simulink model "W06_P3_boat_speed"  (R2024b)
settings: Solver=ode4  StartTime=0.0  StopTime=60  FixedStep=0.01  RelTol=1e-3
values from neighbouring files (symbols this model uses):
  Kb_u = 2    [W06_pid_setup.m]
  Kd_u = 0    [W06_pid_setup.m]
  Ki_u = 300    [W06_pid_setup.m]    (also in W06_setup.m = 100; W08_setup.m = 100)
  Kp_u = 300    [W06_pid_setup.m]    (also in W06_setup.m; W08_setup.m)
  Nf_u = 20    [W06_pid_setup.m]
  tau_m = 0.30    (= 0.3)    [W06_pid_setup.m]
  X_max = 500    [W06_pid_setup.m]
settings Model: Creator=admin  LastModifiedBy=admin

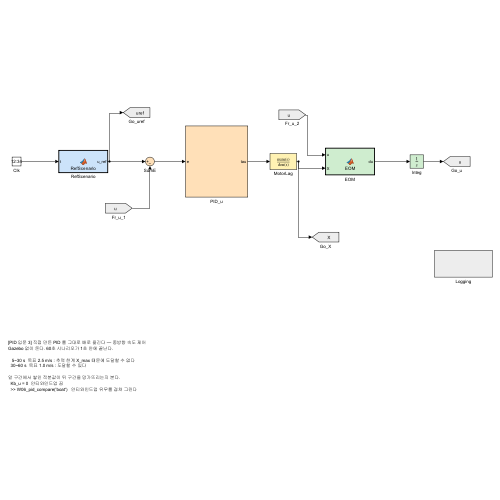
[thumbnail: Simulink's stored preview of the top-level diagram]
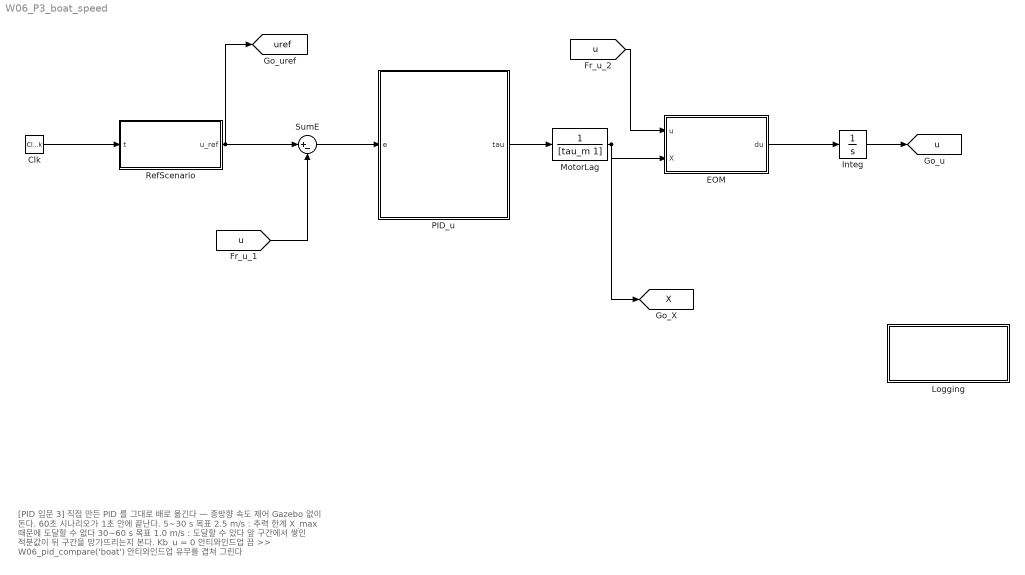
== system W06_P3_boat_speed ==
  note: [PID 입문 3] 직접 만든 PID 를 그대로 배로 옮긴다 — 종방향 속도 제어
      | Gazebo 없이 돈다. 60초 시나리오가 1초 안에 끝난다.
      |
      |    5~30 s  목표 2.5 m/s : 추력 한계 X_max 때문에 도달할 수 없다
      |   30~60 s  목표 1.0 m/s : 도달할 수 있다
      |
      | 앞 구간에서 쌓인 적분값이 뒤 구간을 망가뜨리는지 본다.
      |   Kb_u = 0  안티와인드업 끔
      |   >> W06_pid_compare('boat')   안티와인드업 유무를 겹쳐 그린다
  Clk : DigitalClock  SampleTime=0.01
  EOM : MATLAB Function  TreatAsAtomicUnit=on
  Integ : Integrator
  Logging : Subsystem
  MotorLag : TransferFcn  Numerator=1  Denominator=[tau_m 1]
  PID_u : Subsystem
  RefScenario : MATLAB Function  TreatAsAtomicUnit=on
  SumE : Sum  Inputs=|+-
  tag scope: X=global, u=global, uref=global
  wires:
  Clk/1 -> RefScenario/1(t)
  RefScenario/1(u_ref) -> SumE/1, [uref]
  SumE/1 -> PID_u/1(e)
  PID_u/1(tau) -> MotorLag/1
  EOM/1(du) -> Integ/1
  Integ/1 -> [u]
  MotorLag/1 -> EOM/2(X), [X]
  [u] -> EOM/1(u)
  [u] -> SumE/2

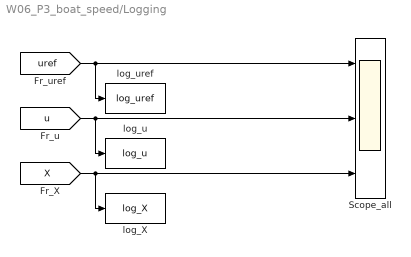
== system W06_P3_boat_speed/Logging ==
  Scope_all : Scope  NumInputPorts=3
  log_X : ToWorkspace  VariableName=log_X  SaveFormat=Timeseries  SampleTime=-1
  log_u : ToWorkspace  VariableName=log_u  SaveFormat=Timeseries  SampleTime=-1
  log_uref : ToWorkspace  VariableName=log_uref  SaveFormat=Timeseries  SampleTime=-1
  wires:
  [uref] -> Scope_all/1, log_uref/1
  [u] -> Scope_all/2, log_u/1
  [X] -> Scope_all/3, log_X/1

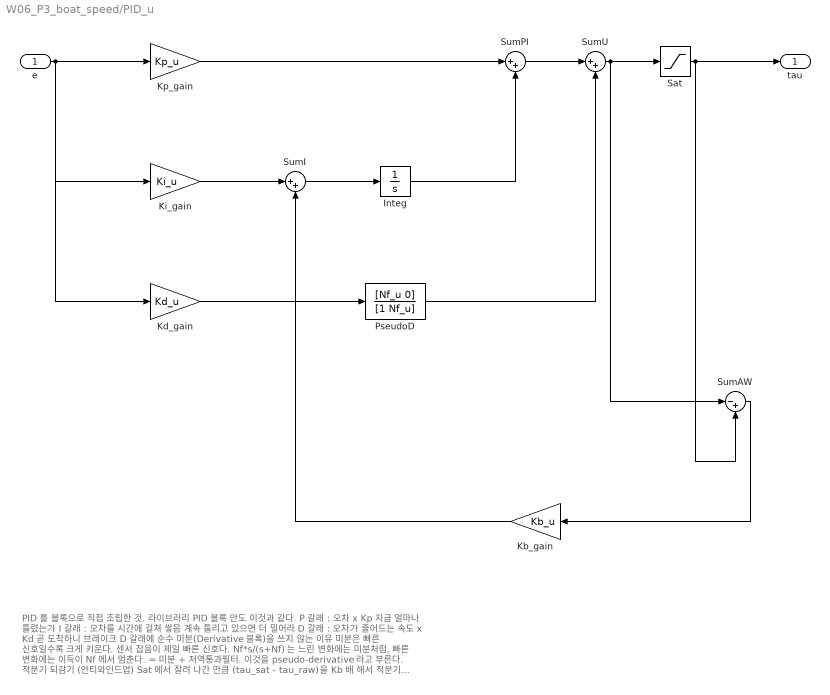
== system W06_P3_boat_speed/PID_u ==
  note: PID 를 블록으로 직접 조립한 것. 라이브러리 PID 블록 안도 이것과 같다.
      |
      |   P 갈래  : 오차 x Kp                        지금 얼마나 틀렸는가
      |   I 갈래  : 오차를 시간에 걸쳐 쌓음            계속 틀리고 있으면 더 밀어라
      |   D 갈래  : 오차가 줄어드는 속도 x Kd          곧 도착하니 브레이크
      |
      | D 갈래에 순수 미분(Derivative 블록)을 쓰지 않는 이유
      |   미분은 빠른 신호일수록 크게 키운다. 센서 잡음이 제일 빠른 신호다.
      |   Nf*s/(s+Nf) 는 느린 변화에는 미분처럼, 빠른 변화에는 이득이 Nf 에서 멈춘다.
      |   = 미분 + 저역통과필터. 이것을 pseudo-derivative 라고 부른다.
      |
      | 적분기 되감기 (안티와인드업)
      |   Sat 에서 잘려 나간 만큼 (tau_sat - tau_raw) 을 Kb 배 해서 적분기 입력에 더한다.
      |   포화 중에는 이 값이 음수라 적분기가 더 쌓이지 못한다.
      |   Kb = 0 으로 두면 되감기가 사라진다. 그것이 와인드업이다.
  e : Inport
  Integ : Integrator
  Kb_gain : Gain  Gain=Kb_u
  Kd_gain : Gain  Gain=Kd_u
  Ki_gain : Gain  Gain=Ki_u
  Kp_gain : Gain  Gain=Kp_u
  PseudoD : TransferFcn  Numerator=[Nf_u 0]  Denominator=[1 Nf_u]
  Sat : Saturate  UpperLimit=X_max  LowerLimit=-X_max
  SumAW : Sum  Inputs=|-+
  SumI : Sum  Inputs=|++
  SumPI : Sum  Inputs=|++
  SumU : Sum  Inputs=|++
  tau : Outport
  wires:
  e/1 -> Kp_gain/1, Ki_gain/1, Kd_gain/1
  Ki_gain/1 -> SumI/1
  SumI/1 -> Integ/1
  Kd_gain/1 -> PseudoD/1
  Kp_gain/1 -> SumPI/1
  SumPI/1 -> SumU/1
  SumU/1 -> Sat/1, SumAW/1
  Sat/1 -> tau/1, SumAW/2
  Integ/1 -> SumPI/2
  PseudoD/1 -> SumU/2
  SumAW/1 -> Kb_gain/1
  Kb_gain/1 -> SumI/2

== matlab function W06_P3_boat_speed/RefScenario ==
  data: t input; u_ref output
function u_ref = RefScenario(t)
%#codegen
% Surge speed command [m/s].
%    0- 5 s : stop
%    5-30 s : 2.5 m/s  -- unreachable. Thrust saturates the whole time
%   30-60 s : 1.0 m/s  -- reachable again
if t < 5
    u_ref = 0;
elseif t < 30
    u_ref = 2.5;
else
    u_ref = 1.0;
end

== matlab function W06_P3_boat_speed/EOM ==
  data: u input; du output; X input
function du = EOM(u, X)
%#codegen
% Surge-only WAM-V equation of motion.
% Same coefficients as W06_5_offline, i.e. the Gazebo VRX plugin.
%   m du/dt = X - (Xu + Xuu*|u|)*u
mm  = 211;
Xu  = 100;
Xuu = 150;
du = (X - (Xu + Xuu*abs(u))*u)/mm;
